simulink model "simulink_ss"  (R2022b)
settings: Solver=VariableStepAuto  StartTime=0.0  StopTime=100  RelTol=1e-3
undefined symbols (not defined in the file): A, B, K, Ki
settings Model: Creator=Omar Wessam  LastModifiedBy=Omar Wessam

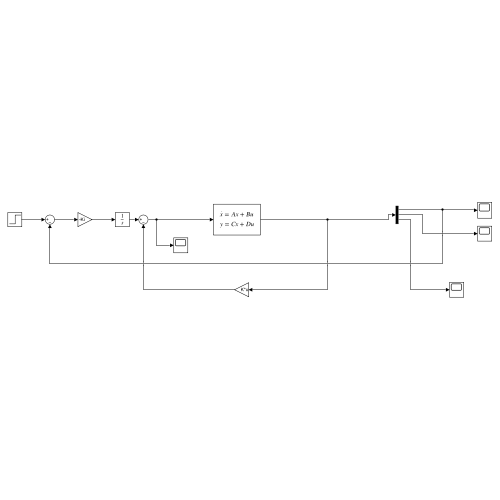
[thumbnail: Simulink's stored preview of the top-level diagram]
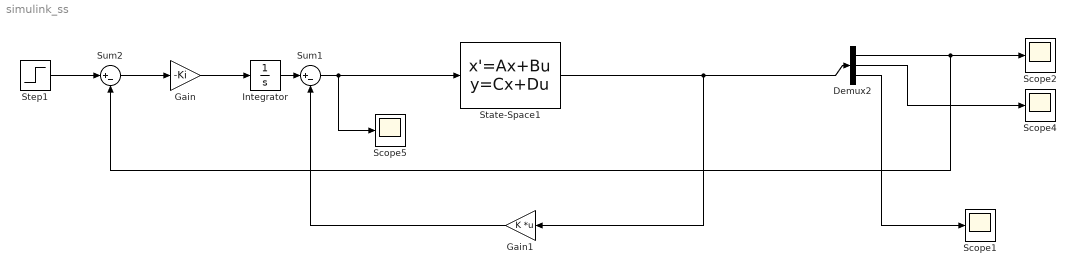
== system simulink_ss ==
  Demux2 : Demux  Outputs=3
  Gain : Gain  Gain=-Ki
  Gain1 : Gain  Gain=K  Multiplication=Matrix(K*u)
  Integrator : Integrator
  Scope{1..2,4..5} (4 alike) : Scope
  State-Space1 : StateSpace  A=A  B=B  C=eye(3)  D=[0;0;0]  InitialCondition=0
  Step1 : Step  Time=-1  After=10  SampleTime=0
  Sum1 : Sum  Inputs=|+-
  Sum2 : Sum  Inputs=|+-
  wires:
  Demux2/1 -> Sum2/2, Scope2/1
  Sum1/1 -> Scope5/1, State-Space1/1
  State-Space1/1 -> Demux2/1, Gain1/1
  Demux2/2 -> Scope4/1
  Gain1/1 -> Sum1/2
  Integrator/1 -> Sum1/1
  Sum2/1 -> Gain/1
  Step1/1 -> Sum2/1
  Demux2/3 -> Scope1/1
  Gain/1 -> Integrator/1
